simulink model "HMIHeightSelc2L"  (R2018b)
settings: Solver=FixedStepDiscrete  StartTime=0.0  StopTime=10.0  RelTol=1e-3
undefined symbols (not defined in the file or in its folder): arg, EEPHMISecRwStPassHeight_Set
settings Model: Creator=sn2xws  LastModifiedBy=sn2xws
settings DataIOCC: SaveFormat=StructureWithTime
settings OptimizationCC: DefaultParameterBehavior=Inlined  EnhancedBackFolding=on  PassReuseOutputArgsAs=Individual arguments  ZeroExternalMemoryAtStartup=off  ZeroInternalMemoryAtStartup=off  OptimizeBlockOrder=speed  DifferentSizesBufferReuse=on  OptimizationCustomize=off
settings DebuggingCC: ParameterTunabilityLossMsg=error
settings SFSimCC: MATLABDynamicMemAlloc=off
settings RTWCC: SystemTargetFile=autosar.tlc  GenCodeOnly=on  TemplateMakefile=ert_default_tmf  Description=AUTOSAR  GenerateReport=on  IncludeHyperlinkInReport=on  LaunchReport=on  GenerateTraceInfo=on  GenerateTraceReport=on  GenerateTraceReportSl=on  GenerateTraceReportSf=on  GenerateTraceReportEml=on  GenerateCodeMetricsReport=on
settings CodeAppCC: ForceParamTrailComments=on  IgnoreCustomStorageClasses=off  OperatorAnnotations=on  SimulinkDataObjDesc=on  SFDataObjDesc=on  InsertBlockDesc=on
settings STFCustomTargetCC: TargetLangStandard=C99 (ISO)  MultiwordLength=256  ParMdlRefBuildCompliant=on  CompOptLevelCompliant=on  IncludeMdlTerminateFcn=off  CombineOutputUpdateFcns=on  SuppressErrorStatus=on  ERTCustomFileBanners=on  SupportNonFinite=off  SupportComplex=off  SupportContinuousTime=off  SupportNonInlinedSFcns=off  RemoveResetFunc=on  MATLABClassNameForMDSCustomization=Simulink.SoftwareTarget.ERTCustomization  AutosarCompliant=on  UseToolchainInfoCompliant=on  LookupTableObjectStructAxisOrder=2,1,3,4,...  LUTObjectStructOrderEvenSpacing=Size,Table,Breakpoints  SystemTargetFile=autosar.tlc
settings ERTTargetCC: TargetLangStandard=C99 (ISO)  ConcurrentExecutionCompliant=off  IncludeMdlTerminateFcn=off  SuppressErrorStatus=on  SupportNonFinite=off  SupportComplex=off  ModelStepFunctionPrototypeControlCompliant=off  CPPClassGenCompliant=off  AutosarCompliant=on  LookupTableObjectStructAxisOrder=2,1,3,4,...  LUTObjectStructOrderEvenSpacing=Size,Table,Breakpoints  InlinedParameterPlacement=NonHierarchical  ERTCustomFileTemplate=example_file_process.tlc  ERTFilePackagingFormat=Compact

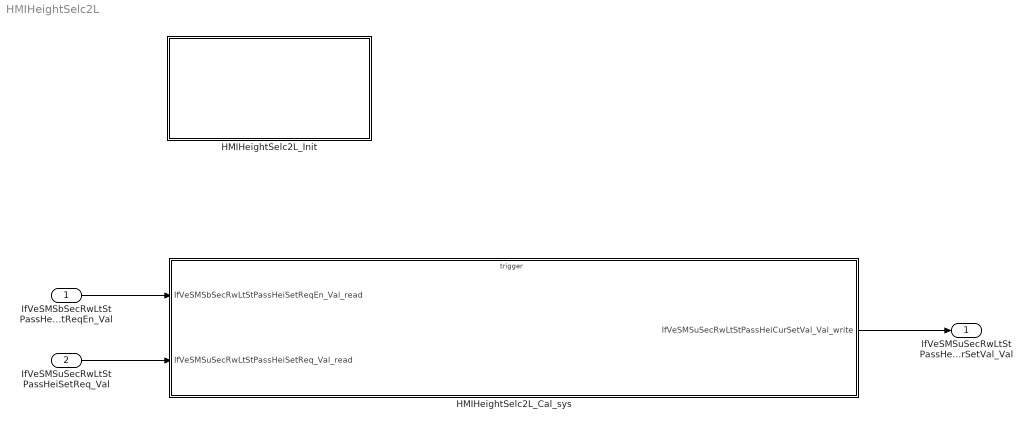
== system HMIHeightSelc2L ==
  IfVeSMSbSecRwLtStPassHeiSetReqEn_Val : Inport  OutDataTypeStr=boolean  PortDimensions=1
  IfVeSMSuSecRwLtStPassHeiSetReq_Val : Inport  Port=2  OutDataTypeStr=uint8  PortDimensions=1
  HMIHeightSelc2L_Cal_sys : Subsystem
  HMIHeightSelc2L_Init : Subsystem
  IfVeSMSuSecRwLtStPassHeiCurSetVal_Val : Outport  OutDataTypeStr=uint8  PortDimensions=1
  wires:
  IfVeSMSbSecRwLtStPassHeiSetReqEn_Val/1 -> HMIHeightSelc2L_Cal_sys/1(IfVeSMSbSecRwLtStPassHeiSetReqEn_Val_read)
  IfVeSMSuSecRwLtStPassHeiSetReq_Val/1 -> HMIHeightSelc2L_Cal_sys/2(IfVeSMSuSecRwLtStPassHeiSetReq_Val_read)
  HMIHeightSelc2L_Cal_sys/1(IfVeSMSuSecRwLtStPassHeiCurSetVal_Val_write) -> IfVeSMSuSecRwLtStPassHeiCurSetVal_Val/1

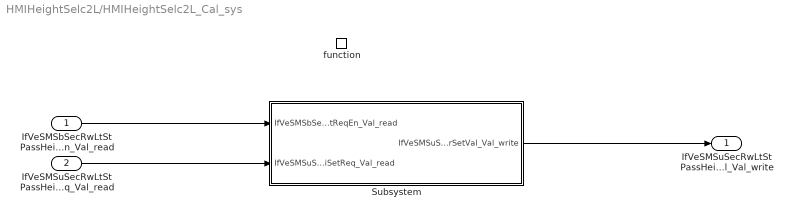
== system HMIHeightSelc2L/HMIHeightSelc2L_Cal_sys ==
  IfVeSMSbSecRwLtStPassHeiSetReqEn_Val_read : Inport
  IfVeSMSuSecRwLtStPassHeiSetReq_Val_read : Inport  Port=2
  function : TriggerPort  TriggerType=function-call  IsSimulinkFunction=on  FunctionName=HMIHeightSelc2L_Cal  VariantControl=(inherit)
  Subsystem : Subsystem
  IfVeSMSuSecRwLtStPassHeiCurSetVal_Val_write : Outport
      settings: EnsureOutportIsVirtual=on
  wires:
  IfVeSMSbSecRwLtStPassHeiSetReqEn_Val_read/1 -> Subsystem/1(IfVeSMSbSecRwLtStPassHeiSetReqEn_Val_read)
  IfVeSMSuSecRwLtStPassHeiSetReq_Val_read/1 -> Subsystem/2(IfVeSMSuSecRwLtStPassHeiSetReq_Val_read)
  Subsystem/1(IfVeSMSuSecRwLtStPassHeiCurSetVal_Val_write) -> IfVeSMSuSecRwLtStPassHeiCurSetVal_Val_write/1

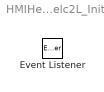
== system HMIHeightSelc2L/HMIHeightSelc2L_Init ==
  Event Listener : EventListener  EventName=reset

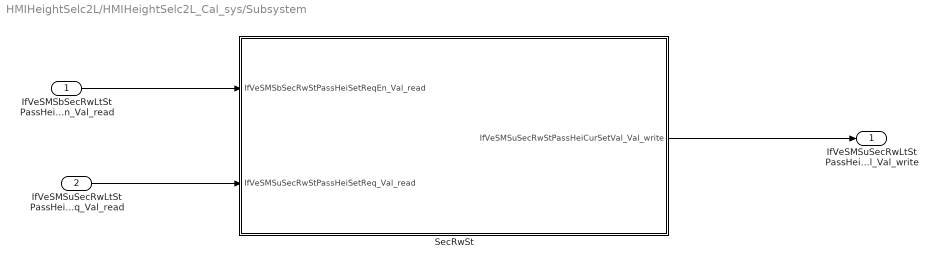
== system HMIHeightSelc2L/HMIHeightSelc2L_Cal_sys/Subsystem ==
  IfVeSMSbSecRwLtStPassHeiSetReqEn_Val_read : Inport
  IfVeSMSuSecRwLtStPassHeiSetReq_Val_read : Inport  Port=2
  SecRwSt : Stateflow chart  TreatAsAtomicUnit=on
  IfVeSMSuSecRwLtStPassHeiCurSetVal_Val_write : Outport
      settings: EnsureOutportIsVirtual=on
  wires:
  IfVeSMSbSecRwLtStPassHeiSetReqEn_Val_read/1 -> SecRwSt/1(IfVeSMSbSecRwStPassHeiSetReqEn_Val_read)
  IfVeSMSuSecRwLtStPassHeiSetReq_Val_read/1 -> SecRwSt/2(IfVeSMSuSecRwStPassHeiSetReq_Val_read)
  SecRwSt/1(IfVeSMSuSecRwStPassHeiCurSetVal_Val_write) -> IfVeSMSuSecRwLtStPassHeiCurSetVal_Val_write/1

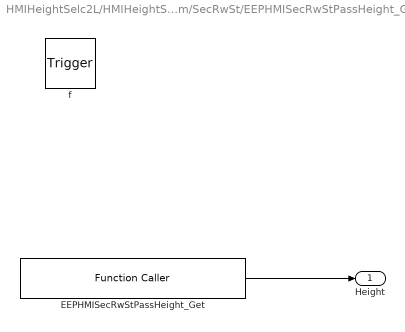
== system HMIHeightSelc2L/HMIHeightSelc2L_Cal_sys/Subsystem/SecRwSt/EEPHMISecRwStPassHeight_Get ==
  f : TriggerPort  TriggerType=function-call  VariantControl=(inherit)
      settings: CopyFcn=Stateflow.SLINSF.SimulinkMan.removeBlockPreDeleteFcn  PreDeleteFcn=Stateflow.SLINSF.SimulinkMan.unsafePredeleteFcn
  EEPHMISecRwStPassHeight_Get : FunctionCaller  FunctionPrototype=arg = EEPHMISecRwStPassHeight_Get()  OutputArgumentSpecifications=P_EEP_Uint8
  Height : Outport
  wires:
  EEPHMISecRwStPassHeight_Get/1 -> Height/1

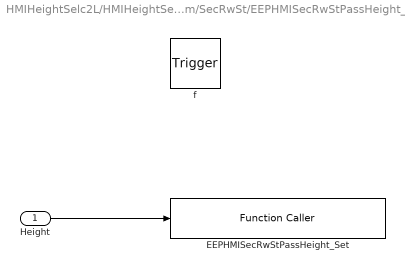
== system HMIHeightSelc2L/HMIHeightSelc2L_Cal_sys/Subsystem/SecRwSt/EEPHMISecRwStPassHeight_Set ==
  Height : Inport
  f : TriggerPort  TriggerType=function-call  VariantControl=(inherit)
      settings: CopyFcn=Stateflow.SLINSF.SimulinkMan.removeBlockPreDeleteFcn  PreDeleteFcn=Stateflow.SLINSF.SimulinkMan.unsafePredeleteFcn
  EEPHMISecRwStPassHeight_Set : FunctionCaller  FunctionPrototype=EEPHMISecRwStPassHeight_Set(arg)  InputArgumentSpecifications=P_EEP_Uint8
  wires:
  Height/1 -> EEPHMISecRwStPassHeight_Set/1

== stateflow chart HMIHeightSelc2L/HMIHeightSelc2L_Cal_sys/Subsystem/SecRwSt ==
  state Height =EEPHMISecRwStPassHeight_Get [function]
  state EEPHMISecRwStPassHeight_Set(Height) [function]
  state SecRwSt
    en:IfVeSMSuSecRwStPassHeiCurSetVal_Val_write = LocalHeight;
    du:IfVeSMSuSecRwStPassHeiCurSetVal_Val_write = LocalHeight;
    state HMIConfig
      en:TmpHeight = IfVeSMSuSecRwStPassHeiSetReq_Val_read;
      du:TmpHeight = IfVeSMSuSecRwStPassHeiSetReq_Val_read;
    state Wait
    state EEPWt
      en:LocalHeight = TmpHeight;
      en:EEPHMISecRwStPassHeight_Set(LocalHeight);
    (default) -> Wait
    Wait -> HMIConfig : [IfVeSMSbSecRwStPassHeiSetReqEn_Val_read]
    (junction 46) -> Wait [order 2]
    HMIConfig -> (junction 46) : [!IfVeSMSbSecRwStPassHeiSetReqEn_Val_read]
    (junction 46) -> (junction 47) [order 1] : [TmpHeight!=LocalHeight]
    EEPWt -> Wait
    (junction 47) -> EEPWt
  (default) -> SecRwSt : {
      | LocalHeight = EEPHMISecRwStPassHeight_Get();
      |  }
  data: Height function_output; Height function_input; IfVeSMSbSecRwStPassHeiSetReqEn_Val_read input; IfVeSMSuSecRwStPassHeiSetReq_Val_read input; IfVeSMSuSecRwStPassHeiCurSetVal_Val_write output; LocalHeight local uint8 =0; TmpHeight local uint8
